simulink model "TypeA_siso180515"  (R2014a)
settings: Solver=ode45  StartTime=0.0  StopTime=12.0  RelTol=1e-3
values from neighbouring files (symbols this model uses):
  gain_actIML = 2.1e-7*1.e+6*20/(2^16)/magIM(inddc)*gain_actIML    [TypeA_reconstruction.m]
  gain_actMNL = 5.1e-6*1.e+6*20/(2^16)/magMN(inddc)*gain_actMNL    [TypeA_reconstruction.m]
  gain_actTML = 1.7e-7*1.e+6*20/(2^16)/magTM(inddc)*gain_actTML    [TypeA_reconstruction.m]
  gainBFL = 0    [main.m]
  gainIPL = 0    [main.m]
  sys1 = sys1_exp    [check_exportvsmake.m]    (also in sumcon2mdlconst_typeA.m = sus.ss)
undefined symbols (not defined in the file or in its folder): cMat_BF, cMat_IM, cMat_MN, cMat_TM, gain_actBFGAS, gain_actBFL, gain_actBFP, gain_actBFR, gain_actBFT, gain_actBFV, gain_actBFY, gain_actF0GAS, gain_actF1GAS, gain_actF2GAS, gain_actF3GAS, gain_actIMP, gain_actIMR, gain_actIMT, gain_actIMV, gain_actIMY, gain_actIPL, gain_actIPT, gain_actIPY, gain_actMNP, gain_actMNR, gain_actMNT, gain_actMNV, gain_actMNY, gain_actTMP, gain_actTMY, gainBFGAS, gainBFP, gainBFR, gainBFT, gainBFV, gainBFY, gainF0GAS, gainF1GAS, gainF2GAS, gainF3GAS, gainHieBFP, gainHieBFR, gainHieBFY, gainHieIML, gainHieIMP, gainHieIMY, gainHieIPL, gainHieIPY, gainHieMNL, gainHieMNP, gainHieMNY, gainIML, gainIMP, gainIMR, gainIMT, gainIMV, gainIMY, gainIPT, gainIPY, gainISC_TML ... (+18)
libraries: cstblocks x57
(part 1 of 2)
settings Model: Creator=kokioktm  LastModifiedBy=ayaka
settings DebuggingCC: MergeDetectMultiDrivingBlocksExec=error  FrameProcessingCompatibilityMsg=error

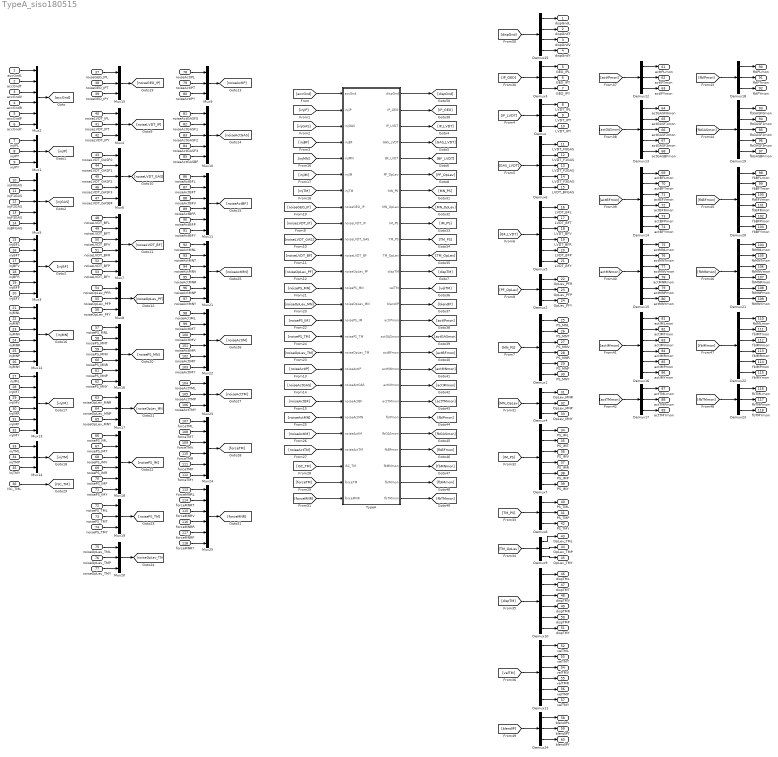
== system TypeA_siso180515 ==
  accGndL : Inport
  accGndT : Inport  Port=2
  accGndV : Inport  Port=3
  accGndR : Inport  Port=4
  accGndP : Inport  Port=5
  accGndY : Inport  Port=6
  injIPL : Inport  Port=7
  injIPT : Inport  Port=8
  injIPY : Inport  Port=9
  injF0GAS : Inport  Port=10
  injF1GAS : Inport  Port=11
  injF2GAS : Inport  Port=12
  injF3GAS : Inport  Port=13
  injBFGAS : Inport  Port=14
  injBFL : Inport  Port=15
  injBFT : Inport  Port=16
  injBFV : Inport  Port=17
  injBFR : Inport  Port=18
  injBFP : Inport  Port=19
  injBFY : Inport  Port=20
  injMNL : Inport  Port=21
  injMNT : Inport  Port=22
  injMNV : Inport  Port=23
  injMNR : Inport  Port=24
  injMNP : Inport  Port=25
  injMNY : Inport  Port=26
  injIML : Inport  Port=27
  injIMT : Inport  Port=28
  injIMV : Inport  Port=29
  injIMR : Inport  Port=30
  injIMP : Inport  Port=31
  injIMY : Inport  Port=32
  injTML : Inport  Port=33
  injTMP : Inport  Port=34
  injTMY : Inport  Port=35
  ISC_TML : Inport  Port=36
  noiseGEO_IPL : Inport  Port=37
  noiseGEO_IPT : Inport  Port=38
  noiseGEO_IPY : Inport  Port=39
  noiseLVDT_IPL : Inport  Port=40
  noiseLVDT_IPT : Inport  Port=41
  noiseLVDT_IPY : Inport  Port=42
  noiseLVDT_GASF0 : Inport  Port=43
  noiseLVDT_GASF1 : Inport  Port=44
  noiseLVDT_GASF2 : Inport  Port=45
  noiseLVDT_GASF3 : Inport  Port=46
  noiseLVDT_GASBF : Inport  Port=47
  noiseLVDT_BFL : Inport  Port=48
  noiseLVDT_BFT : Inport  Port=49
  noiseLVDT_BFV : Inport  Port=50
  noiseLVDT_BFR : Inport  Port=51
  noiseLVDT_BFP : Inport  Port=52
  noiseLVDT_BFY : Inport  Port=53
  noiseOpLev_PFR : Inport  Port=54
  noiseOpLev_PFP : Inport  Port=55
  noiseOpLev_PFY : Inport  Port=56
  noisePS_MNL : Inport  Port=57
  noisePS_MNT : Inport  Port=58
  noisePS_MNV : Inport  Port=59
  noisePS_MNR : Inport  Port=60
  noisePS_MNP : Inport  Port=61
  noisePS_MNY : Inport  Port=62
  noiseOpLev_MNR : Inport  Port=63
  noiseOpLev_MNP : Inport  Port=64
  noiseOpLev_MNY : Inport  Port=65
  noisePS_IML : Inport  Port=66
  noisePS_IMT : Inport  Port=67
  noisePS_IMV : Inport  Port=68
  noisePS_IMR : Inport  Port=69
  noisePS_IMP : Inport  Port=70
  noisePS_IMY : Inport  Port=71
  noisePS_TML : Inport  Port=72
  noisePS_TMT : Inport  Port=73
  noisePS_TMY : Inport  Port=74
  noiseOpLev_TML : Inport  Port=75
  noiseOpLev_TMP : Inport  Port=76
  noiseOpLev_TMY : Inport  Port=77
  noiseActIPL : Inport  Port=78
  noiseActIPT : Inport  Port=79
  noiseActIPY : Inport  Port=80
  noiseActGASF0 : Inport  Port=81
  noiseActGASF1 : Inport  Port=82
  noiseActGASF2 : Inport  Port=83
  noiseActGASF3 : Inport  Port=84
  noiseActGASBF : Inport  Port=85
  noiseActBFL : Inport  Port=86
  noiseActBFT : Inport  Port=87
  noiseActBFV : Inport  Port=88
  noiseActBFR : Inport  Port=89
  noiseActBFP : Inport  Port=90
  noiseActBFY : Inport  Port=91
  noiseActMNL : Inport  Port=92
  noiseActMNT : Inport  Port=93
  noiseActMNV : Inport  Port=94
  noiseActMNR : Inport  Port=95
  noiseActMNP : Inport  Port=96
  noiseActMNY : Inport  Port=97
  noiseActIML : Inport  Port=98
  noiseActIMT : Inport  Port=99
  noiseActIMV : Inport  Port=100
  noiseActIMR : Inport  Port=101
  noiseActIMP : Inport  Port=102
  noiseActIMY : Inport  Port=103
  noiseActTML : Inport  Port=104
  noiseActTMP : Inport  Port=105
  noiseActTMY : Inport  Port=106
  forceTML : Inport  Port=107
  forceTMT : Inport  Port=108
  forceTMV : Inport  Port=109
  forceTMR : Inport  Port=110
  forceTMP : Inport  Port=111
  forceTMY : Inport  Port=112
  forceMNRL : Inport  Port=113
  forceMNRT : Inport  Port=114
  forceMNRV : Inport  Port=115
  forceMNRR : Inport  Port=116
  forceMNRP : Inport  Port=117
  forceMNRY : Inport  Port=118
  Demux{,2..4,8..9,12,17..18,23..24} (11 alike) : Demux  Outputs=3
  Demux{1,5,7,10..11,14..16,20..22} (11 alike) : Demux  Outputs=6
  Demux13 : Demux  Outputs=5
  Demux19 : Demux  Outputs=5
  Demux25 : Demux
  Demux6 : Demux  Outputs=5
  Mux{1,4,8..9,14..15,17,19..20,23} (10 alike) : Mux  Inputs=3
  Mux10 : Mux  Inputs=5
  Mux{2..3,7,11..13,16,18,21..22,24..25} (12 alike) : Mux  Inputs=6
  Mux5 : Mux  Inputs=5
  Mux6 : Mux  Inputs=5
  TypeA : Subsystem
  dispGndL : Outport
  dispGndT : Outport  Port=2
  dispGndV : Outport  Port=3
  dispGndY : Outport  Port=4
  GEO_IPL : Outport  Port=5
  GEO_IPT : Outport  Port=6
  GEO_IPY : Outport  Port=7
  LVDT_IPL : Outport  Port=8
  LVDT_IPT : Outport  Port=9
  LVDT_IPY : Outport  Port=10
  LVDT_F0GAS : Outport  Port=11
  LVDT_F1GAS : Outport  Port=12
  LVDT_F2GAS : Outport  Port=13
  LVDT_F3GAS : Outport  Port=14
  LVDT_BFGAS : Outport  Port=15
  LVDT_BFL : Outport  Port=16
  LVDT_BFT : Outport  Port=17
  LVDT_BFV : Outport  Port=18
  LVDT_BFR : Outport  Port=19
  LVDT_BFP : Outport  Port=20
  LVDT_BFY : Outport  Port=21
  OpLev_PFR : Outport  Port=22
  OpLev_PFP : Outport  Port=23
  OpLev_PFY : Outport  Port=24
  PS_MNL : Outport  Port=25
  PS_MNT : Outport  Port=26
  PS_MNV : Outport  Port=27
  PS_MNR : Outport  Port=28
  PS_MNP : Outport  Port=29
  PS_MNY : Outport  Port=30
  OpLev_MNR : Outport  Port=31
  OpLev_MNP : Outport  Port=32
  OpLev_MNY : Outport  Port=33
  PS_IML : Outport  Port=34
  PS_IMT : Outport  Port=35
  PS_IMV : Outport  Port=36
  PS_IMR : Outport  Port=37
  PS_IMP : Outport  Port=38
  PS_IMY : Outport  Port=39
  PS_TML : Outport  Port=40
  PS_TMP : Outport  Port=41
  PS_TMY : Outport  Port=42
  OpLev_TML : Outport  Port=43
  OpLev_TMP : Outport  Port=44
  OpLev_TMY : Outport  Port=45
  dispTML : Outport  Port=46
  dispTMT : Outport  Port=47
  dispTMV : Outport  Port=48
  dispTMR : Outport  Port=49
  dispTMP : Outport  Port=50
  dispTMY : Outport  Port=51
  velTML : Outport  Port=52
  velTMT : Outport  Port=53
  velTMV : Outport  Port=54
  velTMR : Outport  Port=55
  velTMP : Outport  Port=56
  velTMY : Outport  Port=57
  blendIPL : Outport  Port=58
  blendIPT : Outport  Port=59
  blendIPY : Outport  Port=60
  actIPLmon : Outport  Port=61
  actIPTmon : Outport  Port=62
  actIPYmon : Outport  Port=63
  actGASF0mon : Outport  Port=64
  actGASF1mon : Outport  Port=65
  actGASF2mon : Outport  Port=66
  actGASF3mon : Outport  Port=67
  actGASBFmon : Outport  Port=68
  actBFLmon : Outport  Port=69
  actBFTmon : Outport  Port=70
  actBFVmon : Outport  Port=71
  actBFRmon : Outport  Port=72
  actBFPmon : Outport  Port=73
  actBFYmon : Outport  Port=74
  actMNLmon : Outport  Port=75
  actMNTmon : Outport  Port=76
  actMNVmon : Outport  Port=77
  actMNRmon : Outport  Port=78
  actMNPmon : Outport  Port=79
  actMNYmon : Outport  Port=80
  actIMLmon : Outport  Port=81
  actIMTmon : Outport  Port=82
  actIMVmon : Outport  Port=83
  actIMRmon : Outport  Port=84
  actIMPmon : Outport  Port=85
  actIMYmon : Outport  Port=86
  actTMLmon : Outport  Port=87
  actTMPmon : Outport  Port=88
  actTMYmon : Outport  Port=89
  fbIPLmon : Outport  Port=90
  fbIPTmon : Outport  Port=91
  fbIPYmon : Outport  Port=92
  fbGASF0mon : Outport  Port=93
  fbGASF1mon : Outport  Port=94
  fbGASF2mon : Outport  Port=95
  fbGASF3mon : Outport  Port=96
  fbGASBFmon : Outport  Port=97
  fbBFLmon : Outport  Port=98
  fbBFTmon : Outport  Port=99
  fbBFVmon : Outport  Port=100
  fbBFRmon : Outport  Port=101
  fbBFPmon : Outport  Port=102
  fbBFYmon : Outport  Port=103
  fbMNLmon : Outport  Port=104
  fbMNTmon : Outport  Port=105
  fbMNVmon : Outport  Port=106
  fbMNRmon : Outport  Port=107
  fbMNPmon : Outport  Port=108
  fbMNYmon : Outport  Port=109
  fbIMLmon : Outport  Port=110
  fbIMTmon : Outport  Port=111
  fbIMVmon : Outport  Port=112
  fbIMRmon : Outport  Port=113
  fbIMPmon : Outport  Port=114
  fbIMYmon : Outport  Port=115
  fbTMLmon : Outport  Port=116
  fbTMPmon : Outport  Port=117
  fbTMYmon : Outport  Port=118
  wires:
  [accGnd] -> TypeA/1(accGnd)
  accGndT/1 -> Mux2/2
  accGndL/1 -> Mux2/1
  accGndV/1 -> Mux2/3
  accGndR/1 -> Mux2/4
  accGndP/1 -> Mux2/5
  accGndY/1 -> Mux2/6
  Mux2/1 -> [accGnd]
  injIPL/1 -> Mux1/1
  injIPT/1 -> Mux1/2
  injIPY/1 -> Mux1/3
  Mux1/1 -> [injIP]
  [injIP] -> TypeA/2(injIP)
  injF0GAS/1 -> Mux5/1
  injF1GAS/1 -> Mux5/2
  injF2GAS/1 -> Mux5/3
  injF3GAS/1 -> Mux5/4
  injBFGAS/1 -> Mux5/5
  Mux5/1 -> [injGAS]
  [injGAS] -> TypeA/3(injGAS)
  injBFT/1 -> Mux3/2
  injBFL/1 -> Mux3/1
  injBFV/1 -> Mux3/3
  injBFR/1 -> Mux3/4
  injBFP/1 -> Mux3/5
  injBFY/1 -> Mux3/6
  Mux3/1 -> [injBF]
  [injBF] -> TypeA/4(injBF)
  TypeA/3(IP_LVDT) -> [IP_LVDT]
  TypeA/4(GAS_LVDT) -> [GAS_LVDT]
  TypeA/5(BF_LVDT) -> [BF_LVDT]
  TypeA/12(dispTM) -> [dispTM]
  TypeA/6(PF_OpLev) -> [PF_OpLev]
  [IP_LVDT] -> Demux/1
  Demux/1 -> LVDT_IPL/1
  Demux/2 -> LVDT_IPT/1
  Demux/3 -> LVDT_IPY/1
  [GAS_LVDT] -> Demux6/1
  Demux6/1 -> LVDT_F0GAS/1
  Demux6/2 -> LVDT_F1GAS/1
  Demux6/3 -> LVDT_F2GAS/1
  Demux6/4 -> LVDT_F3GAS/1
  Demux6/5 -> LVDT_BFGAS/1
  [BF_LVDT] -> Demux5/1
  Demux5/1 -> LVDT_BFL/1
  Demux5/2 -> LVDT_BFT/1
  Demux5/3 -> LVDT_BFV/1
  Demux5/4 -> LVDT_BFR/1
  Demux5/5 -> LVDT_BFP/1
  Demux5/6 -> LVDT_BFY/1
  Demux1/1 -> PS_MNL/1
  Demux1/2 -> PS_MNT/1
  Demux1/3 -> PS_MNV/1
  Demux1/4 -> PS_MNR/1
  Demux1/5 -> PS_MNP/1
  Demux1/6 -> PS_MNY/1
  [MN_PS] -> Demux1/1
  [PF_OpLev] -> Demux2/1
  Demux2/2 -> OpLev_PFP/1
  Demux2/3 -> OpLev_PFY/1
  noiseLVDT_IPL/1 -> Mux4/1
  noiseLVDT_IPT/1 -> Mux4/2
  noiseLVDT_IPY/1 -> Mux4/3
  Mux4/1 -> [noiseLVDT_IP]
  noiseLVDT_GASF0/1 -> Mux6/1
  noiseLVDT_GASF1/1 -> Mux6/2
  noiseLVDT_GASF2/1 -> Mux6/3
  noiseLVDT_GASF3/1 -> Mux6/4
  noiseLVDT_GASBF/1 -> Mux6/5
  Mux6/1 -> [noiseLVDT_GAS]
  noiseLVDT_BFT/1 -> Mux7/2
  noiseLVDT_BFL/1 -> Mux7/1
  noiseLVDT_BFV/1 -> Mux7/3
  noiseLVDT_BFR/1 -> Mux7/4
  noiseLVDT_BFP/1 -> Mux7/5
  noiseLVDT_BFY/1 -> Mux7/6
  Mux7/1 -> [noiseLVDT_BF]
  noiseOpLev_PFR/1 -> Mux8/1
  noiseOpLev_PFP/1 -> Mux8/2
  Mux8/1 -> [noiseOpLev_PF]
  [noiseLVDT_IP] -> TypeA/9(noiseLVDT_IP)
  [noiseLVDT_GAS] -> TypeA/10(noiseLVDT_GAS)
  [noiseOpLev_PF] -> TypeA/12(noiseOpLev_PF)
  [noiseLVDT_BF] -> TypeA/11(noiseLVDT_BF)
  noiseActIPL/1 -> Mux9/1
  noiseActIPT/1 -> Mux9/2
  noiseActIPY/1 -> Mux9/3
  Mux9/1 -> [noiseActIP]
  noiseActGASF0/1 -> Mux10/1
  noiseActGASF1/1 -> Mux10/2
  noiseActGASF2/1 -> Mux10/3
  noiseActGASF3/1 -> Mux10/4
  noiseActGASBF/1 -> Mux10/5
  Mux10/1 -> [noiseActGAS]
  noiseActBFT/1 -> Mux11/2
  noiseActBFL/1 -> Mux11/1
  noiseActBFV/1 -> Mux11/3
  noiseActBFR/1 -> Mux11/4
  noiseActBFP/1 -> Mux11/5
  noiseActBFY/1 -> Mux11/6
  Mux11/1 -> [noiseActBF]
  [noiseActGAS] -> TypeA/19(noiseActGAS)
  [noiseActBF] -> TypeA/20(noiseActBF)
  [noiseActIP] -> TypeA/18(noiseActIP)
  [injMN] -> TypeA/5(injMN)
  [injTM] -> TypeA/7(injTM)
  [injIM] -> TypeA/6(injIM)
  injMNT/1 -> Mux12/2
  injMNL/1 -> Mux12/1
  injMNV/1 -> Mux12/3
  injMNR/1 -> Mux12/4
  injMNP/1 -> Mux12/5
  injMNY/1 -> Mux12/6
  Mux12/1 -> [injMN]
  injIMT/1 -> Mux13/2
  injIML/1 -> Mux13/1
  injIMV/1 -> Mux13/3
  injIMR/1 -> Mux13/4
  injIMP/1 -> Mux13/5
  injIMY/1 -> Mux13/6
  Mux13/1 -> [injIM]
  injTML/1 -> Mux14/1
  injTMP/1 -> Mux14/2
  injTMY/1 -> Mux14/3
  Mux14/1 -> [injTM]
  noiseGEO_IPL/1 -> Mux15/1
  noiseGEO_IPT/1 -> Mux15/2
  noiseGEO_IPY/1 -> Mux15/3
  Mux15/1 -> [noiseGEO_IP]
  [noiseGEO_IP] -> TypeA/8(noiseGEO_IP)
  noiseOpLev_PFY/1 -> Mux8/3
  noisePS_MNT/1 -> Mux16/2
  noisePS_MNL/1 -> Mux16/1
  noisePS_MNV/1 -> Mux16/3
  noisePS_MNR/1 -> Mux16/4
  noisePS_MNP/1 -> Mux16/5
  noisePS_MNY/1 -> Mux16/6
  Mux16/1 -> [noisePS_MN]
  noiseOpLev_MNR/1 -> Mux17/1
  noiseOpLev_MNP/1 -> Mux17/2
  Mux17/1 -> [noiseOpLev_MN]
  noiseOpLev_MNY/1 -> Mux17/3
  noisePS_IMT/1 -> Mux18/2
  noisePS_IML/1 -> Mux18/1
  noisePS_IMV/1 -> Mux18/3
  noisePS_IMR/1 -> Mux18/4
  noisePS_IMP/1 -> Mux18/5
  noisePS_IMY/1 -> Mux18/6
  Mux18/1 -> [noisePS_IM]
  noisePS_TML/1 -> Mux19/1
  noisePS_TMT/1 -> Mux19/2
  Mux19/1 -> [noisePS_TM]
  noisePS_TMY/1 -> Mux19/3
  noiseOpLev_TMP/1 -> Mux20/2
  noiseOpLev_TMY/1 -> Mux20/3
  Mux20/1 -> [noiseOpLev_TM]
  [noisePS_MN] -> TypeA/13(noisePS_MN)
  [noisePS_IM] -> TypeA/15(noisePS_IM)
  [noiseOpLev_MN] -> TypeA/14(noiseOpLev_MN)
  [noisePS_TM] -> TypeA/16(noisePS_TM)
  [noiseOpLev_TM] -> TypeA/17(noiseOpLev_TM)
  noiseActMNT/1 -> Mux21/2
  noiseActMNL/1 -> Mux21/1
  noiseActMNV/1 -> Mux21/3
  noiseActMNR/1 -> Mux21/4
  noiseActMNP/1 -> Mux21/5
  noiseActMNY/1 -> Mux21/6
  Mux21/1 -> [noiseActMN]
  noiseActIMT/1 -> Mux22/2
  noiseActIML/1 -> Mux22/1
  noiseActIMV/1 -> Mux22/3
  noiseActIMR/1 -> Mux22/4
  noiseActIMP/1 -> Mux22/5
  noiseActIMY/1 -> Mux22/6
  Mux22/1 -> [noiseActIM]
  noiseActTML/1 -> Mux23/1
  noiseActTMP/1 -> Mux23/2
  noiseActTMY/1 -> Mux23/3
  Mux23/1 -> [noiseActTM]
  forceTMT/1 -> Mux24/2
  forceTML/1 -> Mux24/1
  forceTMV/1 -> Mux24/3
  forceTMR/1 -> Mux24/4
  forceTMP/1 -> Mux24/5
  forceTMY/1 -> Mux24/6
  Mux24/1 -> [forceTM]
  ISC_TML/1 -> [ISC_TM]
  [noiseActMN] -> TypeA/21(noiseActMN)
  [noiseActTM] -> TypeA/23(noiseActTM)
  [noiseActIM] -> TypeA/22(noiseActIM)
  [forceTM] -> TypeA/25(forceTM)
  [ISC_TM] -> TypeA/24(ISC_TM)
  [IP_GEO] -> Demux3/1
  Demux3/1 -> GEO_IPL/1
  Demux3/2 -> GEO_IPT/1
  Demux3/3 -> GEO_IPY/1
  TypeA/2(IP_GEO) -> [IP_GEO]
  Demux2/1 -> OpLev_PFR/1
  TypeA/9(IM_PS) -> [IM_PS]
  TypeA/10(TM_PS) -> [TM_PS]
  TypeA/8(MN_OpLev) -> [MN_OpLev]
  TypeA/7(MN_PS) -> [MN_PS]
  TypeA/11(TM_OpLev) -> [TM_OpLev]
  TypeA/22(fbGASmon) -> [fbGASmon]
  TypeA/16(actGASmon) -> [actGASmon]
  TypeA/21(fbIPmon) -> [fbIPmon]
  TypeA/26(fbTMmon) -> [fbTMmon]
  TypeA/24(fbMNmon) -> [fbMNmon]
  TypeA/15(actIPmon) -> [actIPmon]
  TypeA/19(actIMmon) -> [actIMmon]
  TypeA/14(blendIP) -> [blendIP]
  TypeA/13(velTM) -> [velTM]
  TypeA/25(fbIMmon) -> [fbIMmon]
  TypeA/18(actMNmon) -> [actMNmon]
  TypeA/20(actTMmon) -> [actTMmon]
  TypeA/17(actBFmon) -> [actBFmon]
  TypeA/23(fbBFmon) -> [fbBFmon]
  [MN_OpLev] -> Demux4/1
  Demux4/2 -> OpLev_MNP/1
  Demux4/3 -> OpLev_MNY/1
  Demux4/1 -> OpLev_MNR/1
  Demux7/1 -> PS_IML/1
  Demux7/2 -> PS_IMT/1
  Demux7/3 -> PS_IMV/1
  Demux7/4 -> PS_IMR/1
  Demux7/5 -> PS_IMP/1
  Demux7/6 -> PS_IMY/1
  [IM_PS] -> Demux7/1
  Demux8/1 -> PS_TML/1
  [TM_PS] -> Demux8/1
  Demux8/2 -> PS_TMP/1
  Demux8/3 -> PS_TMY/1
  [TM_OpLev] -> Demux9/1
  Demux10/1 -> dispTML/1
  Demux10/2 -> dispTMT/1
  Demux10/3 -> dispTMV/1
  Demux10/4 -> dispTMR/1
  Demux10/5 -> dispTMP/1
  Demux10/6 -> dispTMY/1
  [dispTM] -> Demux10/1
  Demux11/1 -> velTML/1
  Demux11/2 -> velTMT/1
  Demux11/3 -> velTMV/1
  Demux11/4 -> velTMR/1
  Demux11/5 -> velTMP/1
  Demux11/6 -> velTMY/1
  [velTM] -> Demux11/1
  [actIPmon] -> Demux12/1
  Demux12/1 -> actIPLmon/1
  Demux12/2 -> actIPTmon/1
  Demux12/3 -> actIPYmon/1
  [actGASmon] -> Demux13/1
  Demux13/1 -> actGASF0mon/1
  Demux13/2 -> actGASF1mon/1
  Demux13/3 -> actGASF2mon/1
  Demux13/4 -> actGASF3mon/1
  Demux13/5 -> actGASBFmon/1
  [actBFmon] -> Demux14/1
  Demux14/1 -> actBFLmon/1
  Demux14/2 -> actBFTmon/1
  Demux14/3 -> actBFVmon/1
  Demux14/4 -> actBFRmon/1
  Demux14/5 -> actBFPmon/1
  Demux14/6 -> actBFYmon/1
  [actMNmon] -> Demux15/1
  Demux15/1 -> actMNLmon/1
  Demux15/2 -> actMNTmon/1
  Demux15/3 -> actMNVmon/1
  Demux15/4 -> actMNRmon/1
  Demux15/5 -> actMNPmon/1
  Demux15/6 -> actMNYmon/1
  [actIMmon] -> Demux16/1
  Demux16/1 -> actIMLmon/1
  Demux16/2 -> actIMTmon/1
  Demux16/3 -> actIMVmon/1
  Demux16/4 -> actIMRmon/1
  Demux16/5 -> actIMPmon/1
  Demux16/6 -> actIMYmon/1
  [actTMmon] -> Demux17/1
  Demux17/2 -> actTMPmon/1
  Demux17/3 -> actTMYmon/1
  Demux17/1 -> actTMLmon/1
  [fbIPmon] -> Demux18/1
  Demux18/1 -> fbIPLmon/1
  Demux18/2 -> fbIPTmon/1
  Demux18/3 -> fbIPYmon/1
  [fbGASmon] -> Demux19/1
  Demux19/1 -> fbGASF0mon/1
  Demux19/2 -> fbGASF1mon/1
  Demux19/3 -> fbGASF2mon/1
  Demux19/4 -> fbGASF3mon/1
  Demux19/5 -> fbGASBFmon/1
  [fbBFmon] -> Demux20/1
  Demux20/1 -> fbBFLmon/1
  Demux20/2 -> fbBFTmon/1
  Demux20/3 -> fbBFVmon/1
  Demux20/4 -> fbBFRmon/1
  Demux20/5 -> fbBFPmon/1
  Demux20/6 -> fbBFYmon/1
  [fbMNmon] -> Demux21/1
  Demux21/1 -> fbMNLmon/1
  Demux21/2 -> fbMNTmon/1
  Demux21/3 -> fbMNVmon/1
  Demux21/4 -> fbMNRmon/1
  Demux21/5 -> fbMNPmon/1
  Demux21/6 -> fbMNYmon/1
  [fbIMmon] -> Demux22/1
  Demux22/1 -> fbIMLmon/1
  Demux22/2 -> fbIMTmon/1
  Demux22/3 -> fbIMVmon/1
  Demux22/4 -> fbIMRmon/1
  Demux22/5 -> fbIMPmon/1
  Demux22/6 -> fbIMYmon/1
  [fbTMmon] -> Demux23/1
  Demux23/2 -> fbTMPmon/1
  Demux23/3 -> fbTMYmon/1
  Demux23/1 -> fbTMLmon/1
  Demux24/1 -> blendIPL/1
  [blendIP] -> Demux24/1
  Demux24/2 -> blendIPT/1
  Demux24/3 -> blendIPY/1
  [dispGnd] -> Demux25/1
  Demux25/1 -> dispGndL/1
  Demux25/2 -> dispGndT/1
  Demux25/3 -> dispGndV/1
  Demux25/4 -> dispGndY/1
  TypeA/1(dispGnd) -> [dispGnd]
  forceMNRR/1 -> Mux25/4
  forceMNRP/1 -> Mux25/5
  forceMNRL/1 -> Mux25/1
  forceMNRT/1 -> Mux25/2
  Mux25/1 -> [forceMNR]
  forceMNRV/1 -> Mux25/3
  forceMNRY/1 -> Mux25/6
  [forceMNR] -> TypeA/26(forceMNR)
  noiseOpLev_TML/1 -> Mux20/1
  Demux9/1 -> OpLev_TML/1
  Demux9/2 -> OpLev_TMP/1
  Demux9/3 -> OpLev_TMY/1

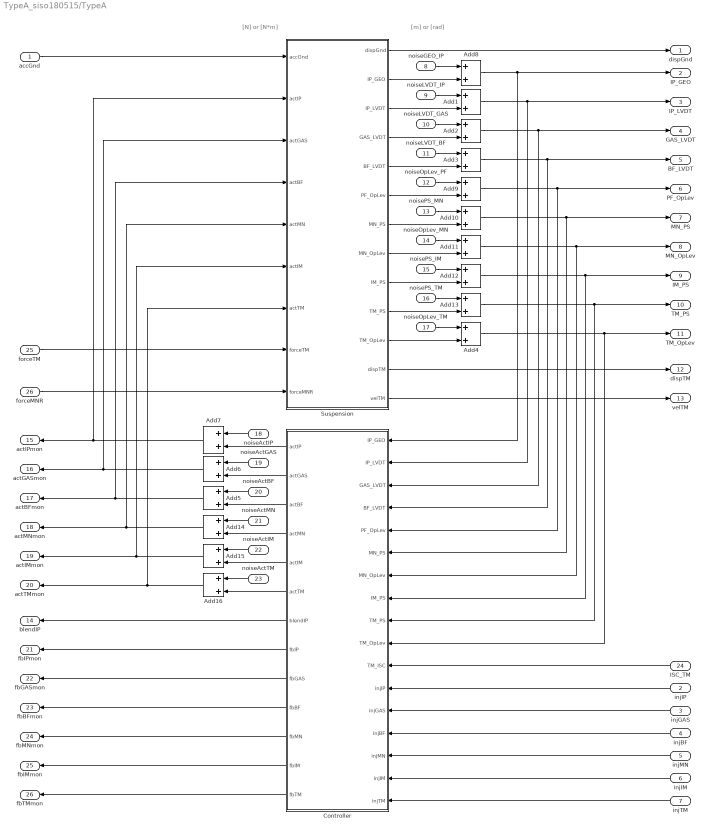
== system TypeA_siso180515/TypeA ==
  note: [N] or [N*m]
  note: [m] or [rad]
  accGnd : Inport
  injIP : Inport  Port=2
  injGAS : Inport  Port=3
  injBF : Inport  Port=4
  injMN : Inport  Port=5
  injIM : Inport  Port=6
  injTM : Inport  Port=7
  noiseGEO_IP : Inport  Port=8
  noiseLVDT_IP : Inport  Port=9
  noiseLVDT_GAS : Inport  Port=10
  noiseLVDT_BF : Inport  Port=11
  noiseOpLev_PF : Inport  Port=12
  noisePS_MN : Inport  Port=13
  noiseOpLev_MN : Inport  Port=14
  noisePS_IM : Inport  Port=15
  noisePS_TM : Inport  Port=16
  noiseOpLev_TM : Inport  Port=17
  noiseActIP : Inport  Port=18
  noiseActGAS : Inport  Port=19
  noiseActBF : Inport  Port=20
  noiseActMN : Inport  Port=21
  noiseActIM : Inport  Port=22
  noiseActTM : Inport  Port=23
  ISC_TM : Inport  Port=24
  forceTM : Inport  Port=25
  forceMNR : Inport  Port=26
  Add{1..16} (16 alike) : Sum
  Controller : Subsystem
  Suspension : Subsystem
  dispGnd : Outport
  IP_GEO : Outport  Port=2
  IP_LVDT : Outport  Port=3
  GAS_LVDT : Outport  Port=4
  BF_LVDT : Outport  Port=5
  PF_OpLev : Outport  Port=6
  MN_PS : Outport  Port=7
  MN_OpLev : Outport  Port=8
  IM_PS : Outport  Port=9
  TM_PS : Outport  Port=10
  TM_OpLev : Outport  Port=11
  dispTM : Outport  Port=12
  velTM : Outport  Port=13
  blendIP : Outport  Port=14
  actIPmon : Outport  Port=15
  actGASmon : Outport  Port=16
  actBFmon : Outport  Port=17
  actMNmon : Outport  Port=18
  actIMmon : Outport  Port=19
  actTMmon : Outport  Port=20
  fbIPmon : Outport  Port=21
  fbGASmon : Outport  Port=22
  fbBFmon : Outport  Port=23
  fbMNmon : Outport  Port=24
  fbIMmon : Outport  Port=25
  fbTMmon : Outport  Port=26
  wires:
  Add1/1 -> IP_LVDT/1, Controller/2(IP_LVDT)
  Add3/1 -> Controller/4(BF_LVDT), BF_LVDT/1
  Add2/1 -> GAS_LVDT/1, Controller/3(GAS_LVDT)
  Suspension/12(dispTM) -> dispTM/1
  Add7/1 -> actIPmon/1, Suspension/2(actIP)
  Add5/1 -> actBFmon/1, Suspension/4(actBF)
  Add4/1 -> Controller/10(TM_OpLev), TM_OpLev/1
  accGnd/1 -> Suspension/1(accGnd)
  Add6/1 -> actGASmon/1, Suspension/3(actGAS)
  injGAS/1 -> Controller/13(injGAS)
  injIP/1 -> Controller/12(injIP)
  injBF/1 -> Controller/14(injBF)
  Controller/10(fbBF) -> fbBFmon/1
  Controller/8(fbIP) -> fbIPmon/1
  Controller/9(fbGAS) -> fbGASmon/1
  Suspension/3(IP_LVDT) -> Add1/2
  Suspension/4(GAS_LVDT) -> Add2/2
  Suspension/5(BF_LVDT) -> Add3/2
  Suspension/11(TM_OpLev) -> Add4/2
  noiseLVDT_IP/1 -> Add1/1
  noiseLVDT_GAS/1 -> Add2/1
  noiseLVDT_BF/1 -> Add3/1
  noiseOpLev_TM/1 -> Add4/1
  Controller/3(actBF) -> Add5/2
  Controller/1(actIP) -> Add7/2
  Controller/2(actGAS) -> Add6/2
  noiseActIP/1 -> Add7/1
  noiseActGAS/1 -> Add6/1
  noiseActBF/1 -> Add5/1
  Add8/1 -> Controller/1(IP_GEO), IP_GEO/1
  noiseGEO_IP/1 -> Add8/1
  Suspension/2(IP_GEO) -> Add8/2
  noiseOpLev_PF/1 -> Add9/1
  Suspension/6(PF_OpLev) -> Add9/2
  Add9/1 -> Controller/5(PF_OpLev), PF_OpLev/1
  noisePS_MN/1 -> Add10/1
  Add10/1 -> Controller/6(MN_PS), MN_PS/1
  noiseOpLev_MN/1 -> Add11/1
  Add11/1 -> Controller/7(MN_OpLev), MN_OpLev/1
  noisePS_IM/1 -> Add12/1
  Add12/1 -> Controller/8(IM_PS), IM_PS/1
  Suspension/8(MN_OpLev) -> Add11/2
  Suspension/7(MN_PS) -> Add10/2
  Suspension/9(IM_PS) -> Add12/2
  noisePS_TM/1 -> Add13/1
  Add13/1 -> Controller/9(TM_PS), TM_PS/1
  Suspension/10(TM_PS) -> Add13/2
  Suspension/13(velTM) -> velTM/1
  injMN/1 -> Controller/15(injMN)
  injTM/1 -> Controller/17(injTM)
  injIM/1 -> Controller/16(injIM)
  ISC_TM/1 -> Controller/11(TM_ISC)
  noiseActMN/1 -> Add14/1
  Add14/1 -> Suspension/5(actMN), actMNmon/1
  Controller/4(actMN) -> Add14/2
  noiseActIM/1 -> Add15/1
  Add15/1 -> Suspension/6(actIM), actIMmon/1
  Controller/5(actIM) -> Add15/2
  noiseActTM/1 -> Add16/1
  Add16/1 -> Suspension/7(actTM), actTMmon/1
  Controller/6(actTM) -> Add16/2
  Controller/7(blendIP) -> blendIP/1
  Controller/13(fbTM) -> fbTMmon/1
  Controller/11(fbMN) -> fbMNmon/1
  Controller/12(fbIM) -> fbIMmon/1
  forceTM/1 -> Suspension/8(forceTM)
  Suspension/1(dispGnd) -> dispGnd/1
  forceMNR/1 -> Suspension/9(forceMNR)

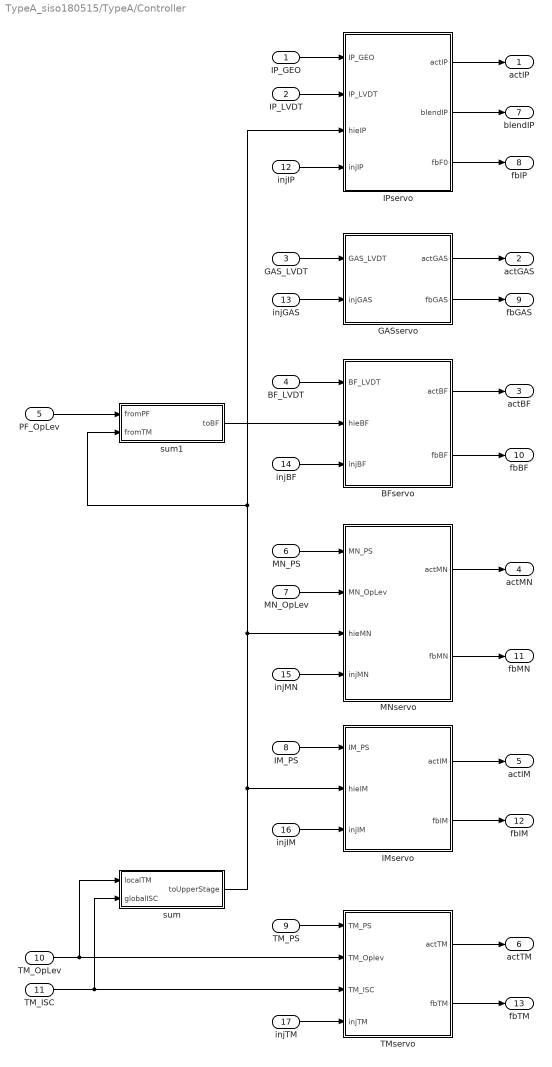
== system TypeA_siso180515/TypeA/Controller ==
  IP_GEO : Inport
  IP_LVDT : Inport  Port=2
  GAS_LVDT : Inport  Port=3
  BF_LVDT : Inport  Port=4
  PF_OpLev : Inport  Port=5
  MN_PS : Inport  Port=6
  MN_OpLev : Inport  Port=7
  IM_PS : Inport  Port=8
  TM_PS : Inport  Port=9
  TM_OpLev : Inport  Port=10
  TM_ISC : Inport  Port=11
  injIP : Inport  Port=12
  injGAS : Inport  Port=13
  injBF : Inport  Port=14
  injMN : Inport  Port=15
  injIM : Inport  Port=16
  injTM : Inport  Port=17
  BFservo : Subsystem
  GASservo : Subsystem
  IMservo : Subsystem
  IPservo : Subsystem
  MNservo : Subsystem
  TMservo : Subsystem
  sum : Subsystem
  sum1 : Subsystem
  actIP : Outport
  actGAS : Outport  Port=2
  actBF : Outport  Port=3
  actMN : Outport  Port=4
  actIM : Outport  Port=5
  actTM : Outport  Port=6
  blendIP : Outport  Port=7
  fbIP : Outport  Port=8
  fbGAS : Outport  Port=9
  fbBF : Outport  Port=10
  fbMN : Outport  Port=11
  fbIM : Outport  Port=12
  fbTM : Outport  Port=13
  wires:
  IP_LVDT/1 -> IPservo/2(IP_LVDT)
  injIP/1 -> IPservo/4(injIP)
  IPservo/3(fbF0) -> fbIP/1
  IPservo/1(actIP) -> actIP/1
  GASservo/1(actGAS) -> actGAS/1
  GASservo/2(fbGAS) -> fbGAS/1
  GAS_LVDT/1 -> GASservo/1(GAS_LVDT)
  injGAS/1 -> GASservo/2(injGAS)
  BF_LVDT/1 -> BFservo/1(BF_LVDT)
  injBF/1 -> BFservo/3(injBF)
  BFservo/1(actBF) -> actBF/1
  BFservo/2(fbBF) -> fbBF/1
  IP_GEO/1 -> IPservo/1(IP_GEO)
  IPservo/2(blendIP) -> blendIP/1
  TM_ISC/1 -> sum/2(globalISC), TMservo/3(TM_ISC)
  TM_OpLev/1 -> sum/1(localTM), TMservo/2(TM_Oplev)
  TM_PS/1 -> TMservo/1(TM_PS)
  injTM/1 -> TMservo/4(injTM)
  MN_PS/1 -> MNservo/1(MN_PS)
  MN_OpLev/1 -> MNservo/2(MN_OpLev)
  injMN/1 -> MNservo/4(injMN)
  IM_PS/1 -> IMservo/1(IM_PS)
  injIM/1 -> IMservo/3(injIM)
  TMservo/1(actTM) -> actTM/1
  TMservo/2(fbTM) -> fbTM/1
  IMservo/2(fbIM) -> fbIM/1
  IMservo/1(actIM) -> actIM/1
  MNservo/2(fbMN) -> fbMN/1
  MNservo/1(actMN) -> actMN/1
  sum/1(toUpperStage) -> sum1/2(fromTM), IPservo/3(hieIP), MNservo/3(hieMN), IMservo/2(hieIM)
  sum1/1(toBF) -> BFservo/2(hieBF)
  PF_OpLev/1 -> sum1/1(fromPF)

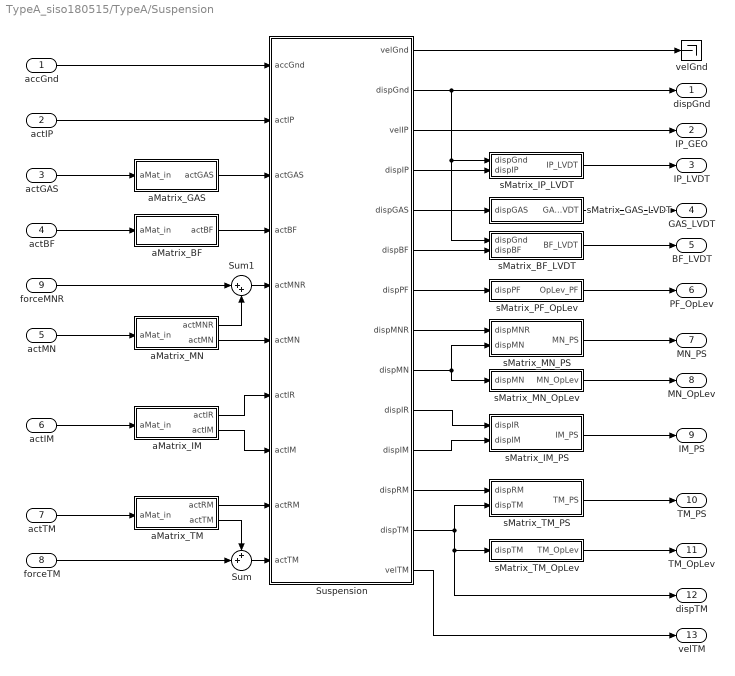
== system TypeA_siso180515/TypeA/Suspension ==
  accGnd : Inport
  actIP : Inport  Port=2
  actGAS : Inport  Port=3
  actBF : Inport  Port=4
  actMN : Inport  Port=5
  actIM : Inport  Port=6
  actTM : Inport  Port=7
  forceTM : Inport  Port=8
  forceMNR : Inport  Port=9
  Sum : Sum  Inputs=++|
  Sum1 : Sum  Inputs=|++
  Suspension : Subsystem
  aMatrix_BF : Subsystem
  aMatrix_GAS : Subsystem
  aMatrix_IM : Subsystem
  aMatrix_MN : Subsystem
  aMatrix_TM : Subsystem
  sMatrix_BF_LVDT : Subsystem
  sMatrix_GAS_LVDT : Subsystem
  sMatrix_IM_PS : Subsystem
  sMatrix_IP_LVDT : Subsystem
  sMatrix_MN_OpLev : Subsystem
  sMatrix_MN_PS : Subsystem
  sMatrix_PF_OpLev : Subsystem
  sMatrix_TM_OpLev : Subsystem
  sMatrix_TM_PS : Subsystem
  velGnd : Terminator
  dispGnd : Outport
  IP_GEO : Outport  Port=2
  IP_LVDT : Outport  Port=3
  GAS_LVDT : Outport  Port=4
  BF_LVDT : Outport  Port=5
  PF_OpLev : Outport  Port=6
  MN_PS : Outport  Port=7
  MN_OpLev : Outport  Port=8
  IM_PS : Outport  Port=9
  TM_PS : Outport  Port=10
  TM_OpLev : Outport  Port=11
  dispTM : Outport  Port=12
  velTM : Outport  Port=13
  wires:
  Suspension/2(dispGnd) -> dispGnd/1, sMatrix_BF_LVDT/1(dispGnd), sMatrix_IP_LVDT/1(dispGnd)
  Suspension/4(dispIP) -> sMatrix_IP_LVDT/2(dispIP)
  Suspension/5(dispGAS) -> sMatrix_GAS_LVDT/1(dispGAS)
  Suspension/6(dispBF) -> sMatrix_BF_LVDT/2(dispBF)
  Suspension/1(velGnd) -> velGnd/1
  sMatrix_IP_LVDT/1(IP_LVDT) -> IP_LVDT/1
  sMatrix_GAS_LVDT/1(GAS_LVDT) -> GAS_LVDT/1
  sMatrix_BF_LVDT/1(BF_LVDT) -> BF_LVDT/1
  Suspension/13(dispTM) -> dispTM/1, sMatrix_TM_OpLev/1(dispTM), sMatrix_TM_PS/2(dispTM)
  accGnd/1 -> Suspension/1(accGnd)
  actIP/1 -> Suspension/2(actIP)
  actGAS/1 -> aMatrix_GAS/1(aMat_in)
  actBF/1 -> aMatrix_BF/1(aMat_in)
  sMatrix_TM_OpLev/1(TM_OpLev) -> TM_OpLev/1
  aMatrix_GAS/1(actGAS) -> Suspension/3(actGAS)
  aMatrix_BF/1(actBF) -> Suspension/4(actBF)
  Suspension/7(dispPF) -> sMatrix_PF_OpLev/1(dispPF)
  sMatrix_PF_OpLev/1(OpLev_PF) -> PF_OpLev/1
  Suspension/8(dispMNR) -> sMatrix_MN_PS/1(dispMNR)
  Suspension/9(dispMN) -> sMatrix_MN_PS/2(dispMN), sMatrix_MN_OpLev/1(dispMN)
  sMatrix_MN_PS/1(MN_PS) -> MN_PS/1
  sMatrix_MN_OpLev/1(MN_OpLev) -> MN_OpLev/1
  Suspension/10(dispIR) -> sMatrix_IM_PS/1(dispIR)
  Suspension/11(dispIM) -> sMatrix_IM_PS/2(dispIM)
  sMatrix_IM_PS/1(IM_PS) -> IM_PS/1
  Suspension/12(dispRM) -> sMatrix_TM_PS/1(dispRM)
  sMatrix_TM_PS/1(TM_PS) -> TM_PS/1
  Suspension/14(velTM) -> velTM/1
  aMatrix_MN/1(actMNR) -> Sum1/2
  aMatrix_MN/2(actMN) -> Suspension/6(actMN)
  actMN/1 -> aMatrix_MN/1(aMat_in)
  actIM/1 -> aMatrix_IM/1(aMat_in)
  aMatrix_IM/1(actIR) -> Suspension/7(actIR)
  aMatrix_IM/2(actIM) -> Suspension/8(actIM)
  actTM/1 -> aMatrix_TM/1(aMat_in)
  aMatrix_TM/1(actRM) -> Suspension/9(actRM)
  Sum/1 -> Suspension/10(actTM)
  aMatrix_TM/2(actTM) -> Sum/1
  forceTM/1 -> Sum/2
  Suspension/3(velIP) -> IP_GEO/1
  Sum1/1 -> Suspension/5(actMNR)
  forceMNR/1 -> Sum1/1

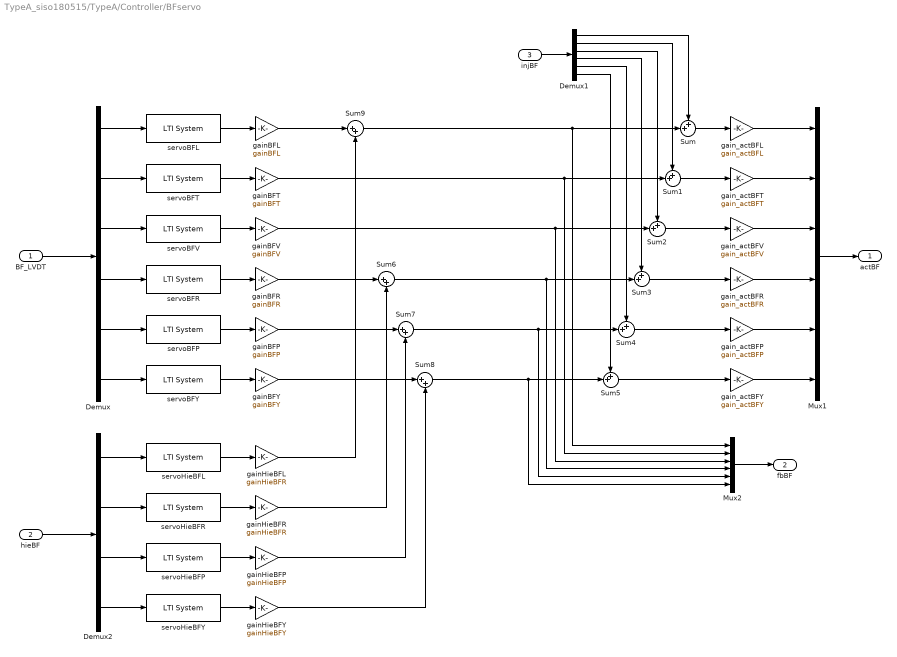
== system TypeA_siso180515/TypeA/Controller/BFservo ==
  BF_LVDT : Inport
  hieBF : Inport  Port=2
  injBF : Inport  Port=3
  Demux : Demux  Outputs=6
  Demux1 : Demux  Outputs=6
  Demux2 : Demux
  Mux1 : Mux  Inputs=6
  Mux2 : Mux  Inputs=6
  Sum{,1..5} (6 alike) : Sum  Inputs=++|
  Sum{6..9} (4 alike) : Sum  Inputs=|++
  gainBFL : Gain  Gain=gainBFL
  gainBFP : Gain  Gain=gainBFP
  gainBFR : Gain  Gain=gainBFR
  gainBFT : Gain  Gain=gainBFT
  gainBFV : Gain  Gain=gainBFV
  gainBFY : Gain  Gain=gainBFY
  gainHieBFL : Gain  Gain=gainHieBFR
  gainHieBFP : Gain  Gain=gainHieBFP
  gainHieBFR : Gain  Gain=gainHieBFR
  gainHieBFY : Gain  Gain=gainHieBFY
  gain_actBFL : Gain  Gain=gain_actBFL
  gain_actBFP : Gain  Gain=gain_actBFP
  gain_actBFR : Gain  Gain=gain_actBFR
  gain_actBFT : Gain  Gain=gain_actBFT
  gain_actBFV : Gain  Gain=gain_actBFV
  gain_actBFY : Gain  Gain=gain_actBFY
  servoBFL : cstblocks/LTI System  sys=servoBFL  IC=[]
  servoBFP : cstblocks/LTI System  sys=servoBFP  IC=[]
  servoBFR : cstblocks/LTI System  sys=servoBFR  IC=[]
  servoBFT : cstblocks/LTI System  sys=servoBFT  IC=[]
  servoBFV : cstblocks/LTI System  sys=servoBFV  IC=[]
  servoBFY : cstblocks/LTI System  sys=servoBFY  IC=[]
  servoHieBFL : cstblocks/LTI System  sys=servoHieBFL  IC=[]
  servoHieBFP : cstblocks/LTI System  sys=servoHieBFP  IC=[]
  servoHieBFR : cstblocks/LTI System  sys=servoHieBFR  IC=[]
  servoHieBFY : cstblocks/LTI System  sys=servoHieBFY  IC=[]
  actBF : Outport
  fbBF : Outport  Port=2
  wires:
  BF_LVDT/1 -> Demux/1
  servoBFL/1 -> gainBFL/1
  servoBFT/1 -> gainBFT/1
  servoBFV/1 -> gainBFV/1
  Demux/1 -> servoBFL/1
  Demux/2 -> servoBFT/1
  Demux/3 -> servoBFV/1
  Sum9/1 -> Sum/2, Mux2/1
  gainBFT/1 -> Sum1/2, Mux2/2
  gainBFV/1 -> Sum2/2, Mux2/3
  injBF/1 -> Demux1/1
  Sum1/1 -> gain_actBFT/1
  Sum2/1 -> gain_actBFV/1
  Sum/1 -> gain_actBFL/1
  Mux1/1 -> actBF/1
  Mux2/1 -> fbBF/1
  Demux1/3 -> Sum2/1
  Demux1/2 -> Sum1/1
  Demux1/1 -> Sum/1
  servoBFR/1 -> gainBFR/1
  servoBFP/1 -> gainBFP/1
  Sum6/1 -> Sum3/2, Mux2/4
  Sum7/1 -> Sum4/2, Mux2/5
  Demux/4 -> servoBFR/1
  Demux/5 -> servoBFP/1
  Demux1/4 -> Sum3/1
  Demux1/5 -> Sum4/1
  Sum3/1 -> gain_actBFR/1
  Sum4/1 -> gain_actBFP/1
  servoBFY/1 -> gainBFY/1
  Sum8/1 -> Sum5/2, Mux2/6
  Demux/6 -> servoBFY/1
  Sum5/1 -> gain_actBFY/1
  Demux1/6 -> Sum5/1
  gain_actBFV/1 -> Mux1/3
  gain_actBFY/1 -> Mux1/6
  gain_actBFR/1 -> Mux1/4
  gain_actBFT/1 -> Mux1/2
  gain_actBFL/1 -> Mux1/1
  gain_actBFP/1 -> Mux1/5
  servoHieBFR/1 -> gainHieBFR/1
  servoHieBFP/1 -> gainHieBFP/1
  servoHieBFY/1 -> gainHieBFY/1
  hieBF/1 -> Demux2/1
  gainBFR/1 -> Sum6/1
  gainBFP/1 -> Sum7/1
  gainBFY/1 -> Sum8/1
  gainHieBFR/1 -> Sum6/2
  gainHieBFP/1 -> Sum7/2
  gainHieBFY/1 -> Sum8/2
  Demux2/1 -> servoHieBFL/1
  Demux2/2 -> servoHieBFR/1
  Demux2/3 -> servoHieBFP/1
  Demux2/4 -> servoHieBFY/1
  servoHieBFL/1 -> gainHieBFL/1
  gainBFL/1 -> Sum9/1
  gainHieBFL/1 -> Sum9/2

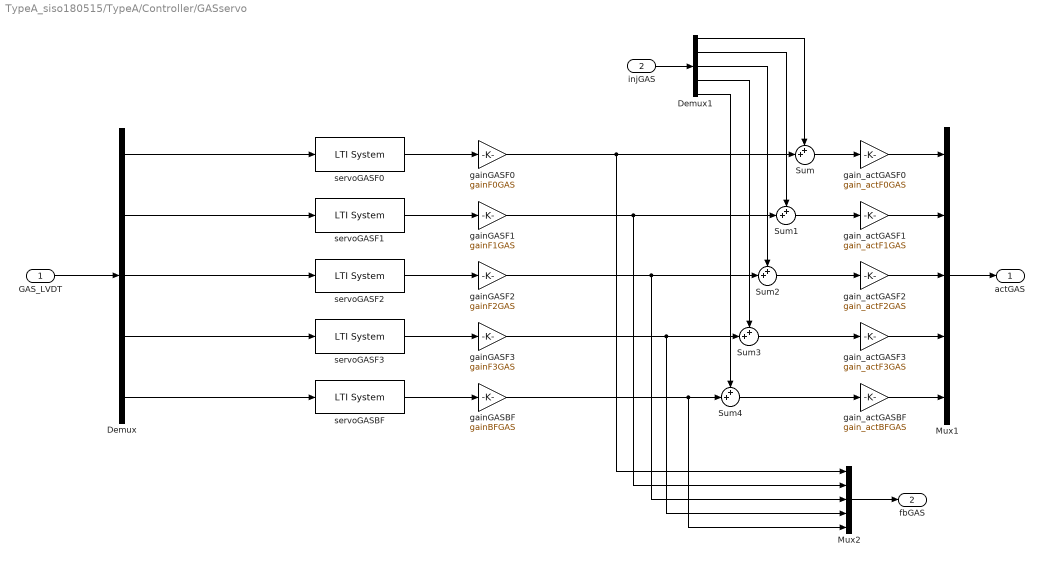
== system TypeA_siso180515/TypeA/Controller/GASservo ==
  GAS_LVDT : Inport
  injGAS : Inport  Port=2
  Demux : Demux  Outputs=5
  Demux1 : Demux  Outputs=5
  Mux1 : Mux  Inputs=5
  Mux2 : Mux  Inputs=5
  Sum{,1..4} (5 alike) : Sum  Inputs=++|
  gainGASBF : Gain  Gain=gainBFGAS
  gainGASF0 : Gain  Gain=gainF0GAS
  gainGASF1 : Gain  Gain=gainF1GAS
  gainGASF2 : Gain  Gain=gainF2GAS
  gainGASF3 : Gain  Gain=gainF3GAS
  gain_actGASBF : Gain  Gain=gain_actBFGAS
  gain_actGASF0 : Gain  Gain=gain_actF0GAS
  gain_actGASF1 : Gain  Gain=gain_actF1GAS
  gain_actGASF2 : Gain  Gain=gain_actF2GAS
  gain_actGASF3 : Gain  Gain=gain_actF3GAS
  servoGASBF : cstblocks/LTI System  sys=servoBFGAS  IC=[]
  servoGASF0 : cstblocks/LTI System  sys=servoF0GAS  IC=[]
  servoGASF1 : cstblocks/LTI System  sys=servoF1GAS  IC=[]
  servoGASF2 : cstblocks/LTI System  sys=servoF2GAS  IC=[]
  servoGASF3 : cstblocks/LTI System  sys=servoF3GAS  IC=[]
  actGAS : Outport
  fbGAS : Outport  Port=2
  wires:
  GAS_LVDT/1 -> Demux/1
  servoGASF0/1 -> gainGASF0/1
  servoGASF1/1 -> gainGASF1/1
  servoGASF2/1 -> gainGASF2/1
  Demux/1 -> servoGASF0/1
  Demux/2 -> servoGASF1/1
  Demux/3 -> servoGASF2/1
  gainGASF0/1 -> Sum/2, Mux2/1
  gainGASF1/1 -> Sum1/2, Mux2/2
  gainGASF2/1 -> Sum2/2, Mux2/3
  injGAS/1 -> Demux1/1
  Sum1/1 -> gain_actGASF1/1
  Sum2/1 -> gain_actGASF2/1
  Sum/1 -> gain_actGASF0/1
  Mux1/1 -> actGAS/1
  Mux2/1 -> fbGAS/1
  Demux1/3 -> Sum2/1
  Demux1/2 -> Sum1/1
  Demux1/1 -> Sum/1
  servoGASF3/1 -> gainGASF3/1
  servoGASBF/1 -> gainGASBF/1
  gainGASF3/1 -> Sum3/2, Mux2/4
  gainGASBF/1 -> Sum4/2, Mux2/5
  Demux/4 -> servoGASF3/1
  Demux/5 -> servoGASBF/1
  Demux1/4 -> Sum3/1
  Demux1/5 -> Sum4/1
  Sum3/1 -> gain_actGASF3/1
  Sum4/1 -> gain_actGASBF/1
  gain_actGASF0/1 -> Mux1/1
  gain_actGASF2/1 -> Mux1/3
  gain_actGASF1/1 -> Mux1/2
  gain_actGASF3/1 -> Mux1/4
  gain_actGASBF/1 -> Mux1/5

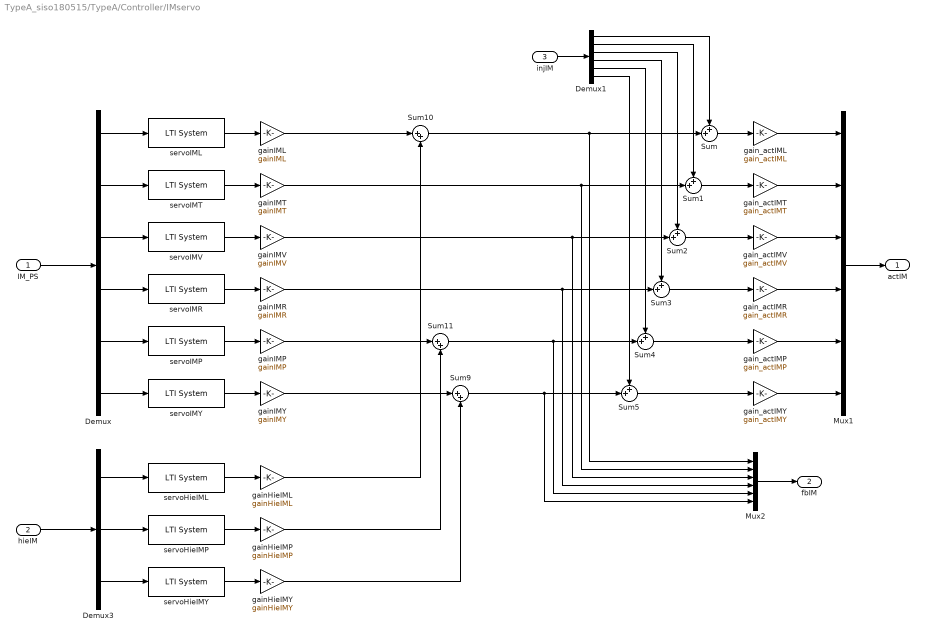
== system TypeA_siso180515/TypeA/Controller/IMservo ==
  IM_PS : Inport
  hieIM : Inport  Port=2
  injIM : Inport  Port=3
  Demux : Demux  Outputs=6
  Demux1 : Demux  Outputs=6
  Demux3 : Demux  Outputs=3
  Mux1 : Mux  Inputs=6
  Mux2 : Mux  Inputs=6
  Sum{,1..5} (6 alike) : Sum  Inputs=++|
  Sum10 : Sum  Inputs=|++
  Sum11 : Sum  Inputs=|++
  Sum9 : Sum  Inputs=|++
  gainHieIML : Gain  Gain=gainHieIML
  gainHieIMP : Gain  Gain=gainHieIMP
  gainHieIMY : Gain  Gain=gainHieIMY
  gainIML : Gain  Gain=gainIML
  gainIMP : Gain  Gain=gainIMP
  gainIMR : Gain  Gain=gainIMR
  gainIMT : Gain  Gain=gainIMT
  gainIMV : Gain  Gain=gainIMV
  gainIMY : Gain  Gain=gainIMY
  gain_actIML : Gain  Gain=gain_actIML
  gain_actIMP : Gain  Gain=gain_actIMP
  gain_actIMR : Gain  Gain=gain_actIMR
  gain_actIMT : Gain  Gain=gain_actIMT
  gain_actIMV : Gain  Gain=gain_actIMV
  gain_actIMY : Gain  Gain=gain_actIMY
  servoHieIML : cstblocks/LTI System  sys=servoHieIML  IC=[]
  servoHieIMP : cstblocks/LTI System  sys=servoHieIMP  IC=[]
  servoHieIMY : cstblocks/LTI System  sys=servoHieIMY  IC=[]
  servoIML : cstblocks/LTI System  sys=servoIML  IC=[]
  servoIMP : cstblocks/LTI System  sys=servoIMP  IC=[]
  servoIMR : cstblocks/LTI System  sys=servoIMR  IC=[]
  servoIMT : cstblocks/LTI System  sys=servoIMT  IC=[]
  servoIMV : cstblocks/LTI System  sys=servoIMV  IC=[]
  servoIMY : cstblocks/LTI System  sys=servoIMY  IC=[]
  actIM : Outport
  fbIM : Outport  Port=2
  wires:
  IM_PS/1 -> Demux/1
  servoIML/1 -> gainIML/1
  servoIMT/1 -> gainIMT/1
  servoIMV/1 -> gainIMV/1
  Demux/1 -> servoIML/1
  Demux/2 -> servoIMT/1
  Demux/3 -> servoIMV/1
  Sum10/1 -> Sum/2, Mux2/1
  gainIMT/1 -> Sum1/2, Mux2/2
  gainIMV/1 -> Sum2/2, Mux2/3
  injIM/1 -> Demux1/1
  Sum1/1 -> gain_actIMT/1
  Sum2/1 -> gain_actIMV/1
  Sum/1 -> gain_actIML/1
  Mux1/1 -> actIM/1
  Mux2/1 -> fbIM/1
  Demux1/3 -> Sum2/1
  Demux1/2 -> Sum1/1
  Demux1/1 -> Sum/1
  servoIMR/1 -> gainIMR/1
  servoIMP/1 -> gainIMP/1
  gainIMR/1 -> Sum3/2, Mux2/4
  Sum11/1 -> Sum4/2, Mux2/5
  Demux/4 -> servoIMR/1
  Demux/5 -> servoIMP/1
  Demux1/4 -> Sum3/1
  Demux1/5 -> Sum4/1
  Sum3/1 -> gain_actIMR/1
  Sum4/1 -> gain_actIMP/1
  servoIMY/1 -> gainIMY/1
  Sum9/1 -> Sum5/2, Mux2/6
  Demux/6 -> servoIMY/1
  Sum5/1 -> gain_actIMY/1
  Demux1/6 -> Sum5/1
  gain_actIMV/1 -> Mux1/3
  gain_actIMY/1 -> Mux1/6
  gain_actIMR/1 -> Mux1/4
  gain_actIMT/1 -> Mux1/2
  gain_actIML/1 -> Mux1/1
  gain_actIMP/1 -> Mux1/5
  servoHieIML/1 -> gainHieIML/1
  servoHieIMP/1 -> gainHieIMP/1
  servoHieIMY/1 -> gainHieIMY/1
  hieIM/1 -> Demux3/1
  Demux3/1 -> servoHieIML/1
  Demux3/2 -> servoHieIMP/1
  Demux3/3 -> servoHieIMY/1
  gainIML/1 -> Sum10/1
  gainIMP/1 -> Sum11/1
  gainHieIML/1 -> Sum10/2
  gainHieIMP/1 -> Sum11/2
  gainHieIMY/1 -> Sum9/2
  gainIMY/1 -> Sum9/1

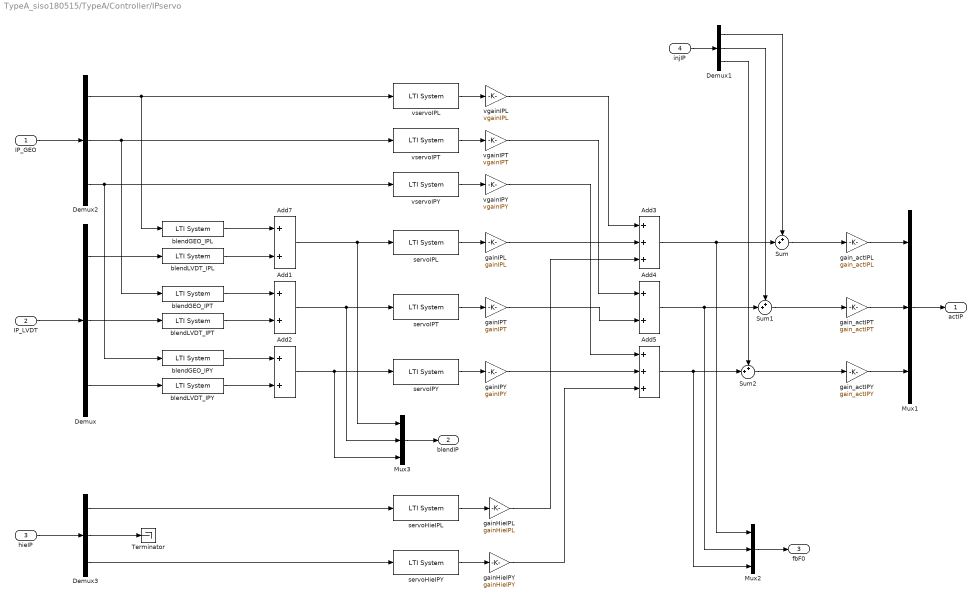
== system TypeA_siso180515/TypeA/Controller/IPservo ==
  IP_GEO : Inport
  IP_LVDT : Inport  Port=2
  hieIP : Inport  Port=3
  injIP : Inport  Port=4
  Add{1..2,4,7} (4 alike) : Sum
  Add3 : Sum  Inputs=+++
  Add5 : Sum  Inputs=+++
  Demux{,1..3} (4 alike) : Demux  Outputs=3
  Mux1 : Mux  Inputs=3
  Mux2 : Mux  Inputs=3
  Mux3 : Mux  Inputs=3
  Sum : Sum  Inputs=++|
  Sum1 : Sum  Inputs=++|
  Sum2 : Sum  Inputs=++|
  Terminator : Terminator
  blendGEO_IPL : cstblocks/LTI System  sys=blendGEO_IPL  IC=[]
  blendGEO_IPT : cstblocks/LTI System  sys=blendGEO_IPT  IC=[]
  blendGEO_IPY : cstblocks/LTI System  sys=blendGEO_IPY  IC=[]
  blendLVDT_IPL : cstblocks/LTI System  sys=blendLVDT_IPL  IC=[]
  blendLVDT_IPT : cstblocks/LTI System  sys=blendLVDT_IPT  IC=[]
  blendLVDT_IPY : cstblocks/LTI System  sys=blendLVDT_IPY  IC=[]
  gainHieIPL : Gain  Gain=gainHieIPL
  gainHieIPY : Gain  Gain=gainHieIPY
  gainIPL : Gain  Gain=gainIPL
  gainIPT : Gain  Gain=gainIPT
  gainIPY : Gain  Gain=gainIPY
  gain_actIPL : Gain  Gain=gain_actIPL
  gain_actIPT : Gain  Gain=gain_actIPT
  gain_actIPY : Gain  Gain=gain_actIPY
  servoHieIPL : cstblocks/LTI System  sys=servoHieIPL  IC=[]
  servoHieIPY : cstblocks/LTI System  sys=servoHieIPY  IC=[]
  servoIPL : cstblocks/LTI System  sys=servoIPL  IC=[]
  servoIPT : cstblocks/LTI System  sys=servoIPT  IC=[]
  servoIPY : cstblocks/LTI System  sys=servoIPY  IC=[]
  vgainIPL : Gain  Gain=vgainIPL
  vgainIPT : Gain  Gain=vgainIPT
  vgainIPY : Gain  Gain=vgainIPY
  vservoIPL : cstblocks/LTI System  sys=vservoIPL  IC=[]
  vservoIPT : cstblocks/LTI System  sys=vservoIPT  IC=[]
  vservoIPY : cstblocks/LTI System  sys=vservoIPY  IC=[]
  actIP : Outport
  blendIP : Outport  Port=2
  fbF0 : Outport  Port=3
  wires:
  IP_LVDT/1 -> Demux/1
  servoIPL/1 -> gainIPL/1
  servoIPT/1 -> gainIPT/1
  servoIPY/1 -> gainIPY/1
  Add3/1 -> Sum/2, Mux2/1
  Add4/1 -> Sum1/2, Mux2/2
  Add5/1 -> Sum2/2, Mux2/3
  injIP/1 -> Demux1/1
  Sum1/1 -> gain_actIPT/1
  Sum2/1 -> gain_actIPY/1
  Sum/1 -> gain_actIPL/1
  Mux1/1 -> actIP/1
  Mux2/1 -> fbF0/1
  Demux1/3 -> Sum2/1
  Demux1/2 -> Sum1/1
  Demux1/1 -> Sum/1
  gain_actIPT/1 -> Mux1/2
  gain_actIPL/1 -> Mux1/1
  gain_actIPY/1 -> Mux1/3
  Demux/2 -> blendLVDT_IPT/1
  Demux/3 -> blendLVDT_IPY/1
  Demux/1 -> blendLVDT_IPL/1
  IP_GEO/1 -> Demux2/1
  Demux2/2 -> vservoIPT/1, blendGEO_IPT/1
  Demux2/3 -> vservoIPY/1, blendGEO_IPY/1
  Demux2/1 -> vservoIPL/1, blendGEO_IPL/1
  Add7/1 -> Mux3/1, servoIPL/1
  Add1/1 -> Mux3/2, servoIPT/1
  Add2/1 -> Mux3/3, servoIPY/1
  blendGEO_IPL/1 -> Add7/1
  blendGEO_IPT/1 -> Add1/1
  blendGEO_IPY/1 -> Add2/1
  blendLVDT_IPL/1 -> Add7/2
  blendLVDT_IPT/1 -> Add1/2
  blendLVDT_IPY/1 -> Add2/2
  Mux3/1 -> blendIP/1
  vservoIPL/1 -> vgainIPL/1
  vservoIPT/1 -> vgainIPT/1
  vservoIPY/1 -> vgainIPY/1
  gainIPY/1 -> Add5/2
  gainIPT/1 -> Add4/2
  gainIPL/1 -> Add3/2
  vgainIPL/1 -> Add3/1
  vgainIPT/1 -> Add4/1
  vgainIPY/1 -> Add5/1
  servoHieIPL/1 -> gainHieIPL/1
  servoHieIPY/1 -> gainHieIPY/1
  hieIP/1 -> Demux3/1
  Demux3/1 -> servoHieIPL/1
  Demux3/3 -> servoHieIPY/1
  gainHieIPL/1 -> Add3/3
  gainHieIPY/1 -> Add5/3
  Demux3/2 -> Terminator/1

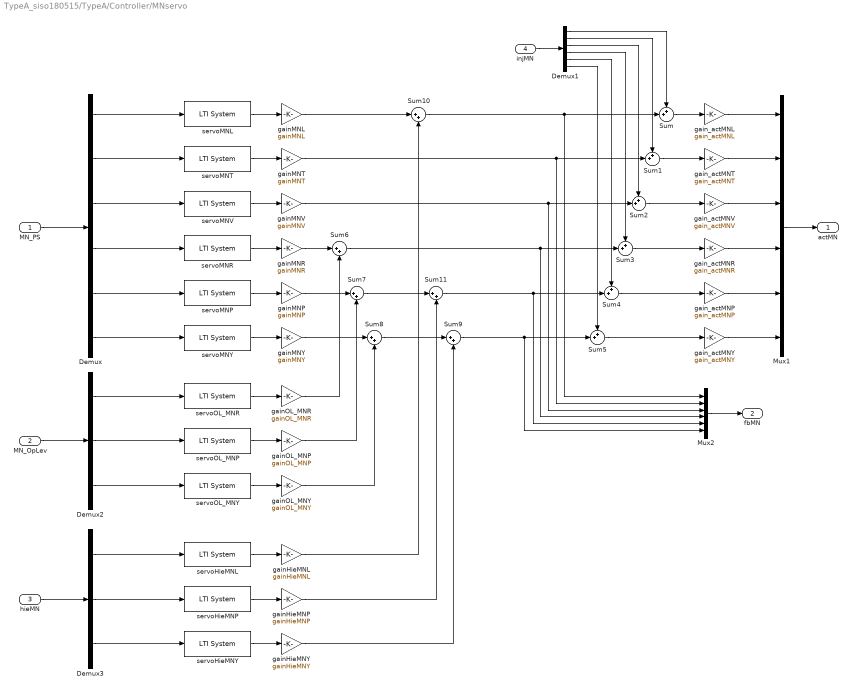
== system TypeA_siso180515/TypeA/Controller/MNservo ==
  MN_PS : Inport
  MN_OpLev : Inport  Port=2
  hieMN : Inport  Port=3
  injMN : Inport  Port=4
  Demux : Demux  Outputs=6
  Demux1 : Demux  Outputs=6
  Demux2 : Demux  Outputs=3
  Demux3 : Demux  Outputs=3
  Mux1 : Mux  Inputs=6
  Mux2 : Mux  Inputs=6
  Sum{,1..5} (6 alike) : Sum  Inputs=++|
  Sum{6..11} (6 alike) : Sum  Inputs=|++
  gainHieMNL : Gain  Gain=gainHieMNL
  gainHieMNP : Gain  Gain=gainHieMNP
  gainHieMNY : Gain  Gain=gainHieMNY
  gainMNL : Gain  Gain=gainMNL
  gainMNP : Gain  Gain=gainMNP
  gainMNR : Gain  Gain=gainMNR
  gainMNT : Gain  Gain=gainMNT
  gainMNV : Gain  Gain=gainMNV
  gainMNY : Gain  Gain=gainMNY
  gainOL_MNP : Gain  Gain=gainOL_MNP
  gainOL_MNR : Gain  Gain=gainOL_MNR
  gainOL_MNY : Gain  Gain=gainOL_MNY
  gain_actMNL : Gain  Gain=gain_actMNL
  gain_actMNP : Gain  Gain=gain_actMNP
  gain_actMNR : Gain  Gain=gain_actMNR
  gain_actMNT : Gain  Gain=gain_actMNT
  gain_actMNV : Gain  Gain=gain_actMNV
  gain_actMNY : Gain  Gain=gain_actMNY
  servoHieMNL : cstblocks/LTI System  sys=servoHieMNL  IC=[]
  servoHieMNP : cstblocks/LTI System  sys=servoHieMNP  IC=[]
  servoHieMNY : cstblocks/LTI System  sys=servoHieMNY  IC=[]
  servoMNL : cstblocks/LTI System  sys=servoMNL  IC=[]
  servoMNP : cstblocks/LTI System  sys=servoMNP  IC=[]
  servoMNR : cstblocks/LTI System  sys=servoMNR  IC=[]
  servoMNT : cstblocks/LTI System  sys=servoMNT  IC=[]
  servoMNV : cstblocks/LTI System  sys=servoMNV  IC=[]
  servoMNY : cstblocks/LTI System  sys=servoMNY  IC=[]
  servoOL_MNP : cstblocks/LTI System  sys=servoOL_MNP  IC=[]
  servoOL_MNR : cstblocks/LTI System  sys=servoOL_MNR  IC=[]
  servoOL_MNY : cstblocks/LTI System  sys=servoOL_MNY  IC=[]
  actMN : Outport
  fbMN : Outport  Port=2
  wires:
  MN_PS/1 -> Demux/1
  servoMNL/1 -> gainMNL/1
  servoMNT/1 -> gainMNT/1
  servoMNV/1 -> gainMNV/1
  Demux/1 -> servoMNL/1
  Demux/2 -> servoMNT/1
  Demux/3 -> servoMNV/1
  Sum10/1 -> Sum/2, Mux2/1
  gainMNT/1 -> Sum1/2, Mux2/2
  gainMNV/1 -> Sum2/2, Mux2/3
  injMN/1 -> Demux1/1
  Sum1/1 -> gain_actMNT/1
  Sum2/1 -> gain_actMNV/1
  Sum/1 -> gain_actMNL/1
  Mux1/1 -> actMN/1
  Mux2/1 -> fbMN/1
  Demux1/3 -> Sum2/1
  Demux1/2 -> Sum1/1
  Demux1/1 -> Sum/1
  servoMNR/1 -> gainMNR/1
  servoMNP/1 -> gainMNP/1
  Sum6/1 -> Sum3/2, Mux2/4
  Sum11/1 -> Sum4/2, Mux2/5
  Demux/4 -> servoMNR/1
  Demux/5 -> servoMNP/1
  Demux1/4 -> Sum3/1
  Demux1/5 -> Sum4/1
  Sum3/1 -> gain_actMNR/1
  Sum4/1 -> gain_actMNP/1
  servoMNY/1 -> gainMNY/1
  Sum9/1 -> Sum5/2, Mux2/6
  Demux/6 -> servoMNY/1
  Sum5/1 -> gain_actMNY/1
  Demux1/6 -> Sum5/1
  gain_actMNV/1 -> Mux1/3
  gain_actMNY/1 -> Mux1/6
  gain_actMNR/1 -> Mux1/4
  gain_actMNT/1 -> Mux1/2
  gain_actMNL/1 -> Mux1/1
  gain_actMNP/1 -> Mux1/5
  servoHieMNL/1 -> gainHieMNL/1
  servoHieMNP/1 -> gainHieMNP/1
  servoHieMNY/1 -> gainHieMNY/1
  servoOL_MNR/1 -> gainOL_MNR/1
  servoOL_MNP/1 -> gainOL_MNP/1
  servoOL_MNY/1 -> gainOL_MNY/1
  MN_OpLev/1 -> Demux2/1
  hieMN/1 -> Demux3/1
  Demux2/1 -> servoOL_MNR/1
  Demux2/2 -> servoOL_MNP/1
  Demux2/3 -> servoOL_MNY/1
  Demux3/1 -> servoHieMNL/1
  gainMNR/1 -> Sum6/1
  gainMNP/1 -> Sum7/1
  gainMNY/1 -> Sum8/1
  gainOL_MNR/1 -> Sum6/2
  gainOL_MNP/1 -> Sum7/2
  gainOL_MNY/1 -> Sum8/2
  gainMNL/1 -> Sum10/1
  Sum7/1 -> Sum11/1
  gainHieMNL/1 -> Sum10/2
  gainHieMNP/1 -> Sum11/2
  gainHieMNY/1 -> Sum9/2
  Sum8/1 -> Sum9/1
  Demux3/2 -> servoHieMNP/1
  Demux3/3 -> servoHieMNY/1

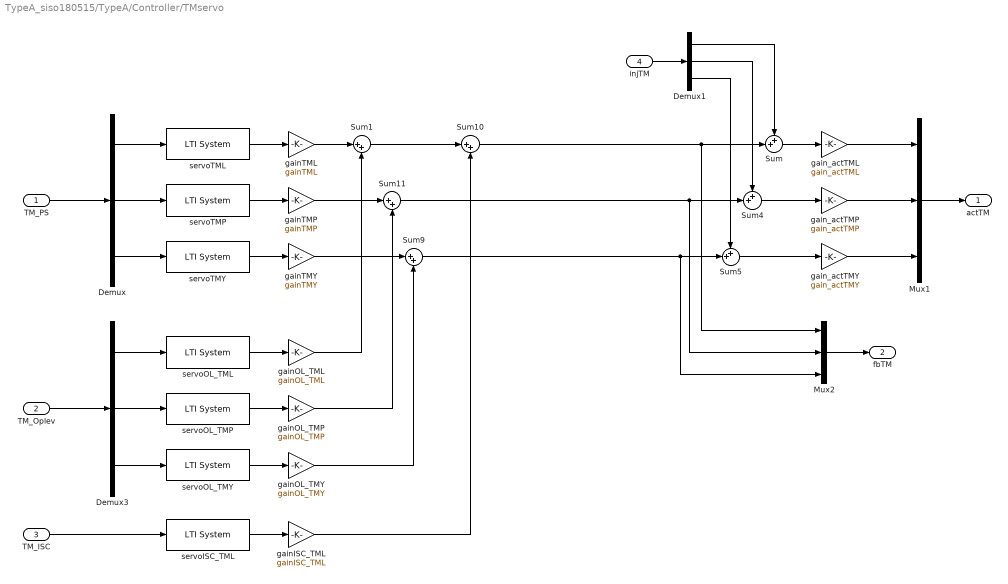
== system TypeA_siso180515/TypeA/Controller/TMservo ==
  TM_PS : Inport
  TM_Oplev : Inport  Port=2
  TM_ISC : Inport  Port=3
  injTM : Inport  Port=4
  Demux : Demux  Outputs=3
  Demux1 : Demux  Outputs=3
  Demux3 : Demux  Outputs=3
  Mux1 : Mux  Inputs=3
  Mux2 : Mux  Inputs=3
  Sum : Sum  Inputs=++|
  Sum{1,9..11} (4 alike) : Sum  Inputs=|++
  Sum4 : Sum  Inputs=++|
  Sum5 : Sum  Inputs=++|
  gainISC_TML : Gain  Gain=gainISC_TML
  gainOL_TML : Gain  Gain=gainOL_TML
  gainOL_TMP : Gain  Gain=gainOL_TMP
  gainOL_TMY : Gain  Gain=gainOL_TMY
  gainTML : Gain  Gain=gainTML
  gainTMP : Gain  Gain=gainTMP
  gainTMY : Gain  Gain=gainTMY
  gain_actTML : Gain  Gain=gain_actTML
  gain_actTMP : Gain  Gain=gain_actTMP
  gain_actTMY : Gain  Gain=gain_actTMY
  servoISC_TML : cstblocks/LTI System  sys=servoISC_TML  IC=[]
  servoOL_TML : cstblocks/LTI System  sys=servoOL_TML  IC=[]
  servoOL_TMP : cstblocks/LTI System  sys=servoOL_TMP  IC=[]
  servoOL_TMY : cstblocks/LTI System  sys=servoOL_TMY  IC=[]
  servoTML : cstblocks/LTI System  sys=servoTML  IC=[]
  servoTMP : cstblocks/LTI System  sys=servoTMP  IC=[]
  servoTMY : cstblocks/LTI System  sys=servoTMY  IC=[]
  actTM : Outport
  fbTM : Outport  Port=2
  wires:
  TM_PS/1 -> Demux/1
  servoTML/1 -> gainTML/1
  Demux/1 -> servoTML/1
  Sum10/1 -> Sum/2, Mux2/1
  injTM/1 -> Demux1/1
  Sum/1 -> gain_actTML/1
  Mux1/1 -> actTM/1
  Mux2/1 -> fbTM/1
  Demux1/1 -> Sum/1
  servoTMP/1 -> gainTMP/1
  Sum11/1 -> Mux2/2, Sum4/2
  Sum4/1 -> gain_actTMP/1
  servoTMY/1 -> gainTMY/1
  Sum9/1 -> Mux2/3, Sum5/2
  Sum5/1 -> gain_actTMY/1
  gain_actTML/1 -> Mux1/1
  servoOL_TMP/1 -> gainOL_TMP/1
  servoOL_TMY/1 -> gainOL_TMY/1
  TM_Oplev/1 -> Demux3/1
  Demux3/2 -> servoOL_TMP/1
  Demux3/3 -> servoOL_TMY/1
  gainTML/1 -> Sum1/1
  gainTMP/1 -> Sum11/1
  gainOL_TMP/1 -> Sum11/2
  gainOL_TMY/1 -> Sum9/2
  gainTMY/1 -> Sum9/1
  Demux/2 -> servoTMP/1
  Demux/3 -> servoTMY/1
  Demux1/2 -> Sum4/1
  Demux1/3 -> Sum5/1
  gain_actTMP/1 -> Mux1/2
  gain_actTMY/1 -> Mux1/3
  servoISC_TML/1 -> gainISC_TML/1
  TM_ISC/1 -> servoISC_TML/1
  gainISC_TML/1 -> Sum10/2
  Demux3/1 -> servoOL_TML/1
  Sum1/1 -> Sum10/1
  gainOL_TML/1 -> Sum1/2
  servoOL_TML/1 -> gainOL_TML/1

== system TypeA_siso180515/TypeA/Controller/sum ==
  localTM : Inport
  globalISC : Inport  Port=2
  Demux4 : Demux  Outputs=3
  Mux3 : Mux  Inputs=3
  Sum : Sum  Inputs=++|
  toUpperStage : Outport
  wires:
  localTM/1 -> Demux4/1
  Mux3/1 -> toUpperStage/1
  Demux4/1 -> Sum/2  "L"
  Demux4/2 -> Mux3/2  "P"
  Demux4/3 -> Mux3/3  "Y"
  globalISC/1 -> Sum/1
  Sum/1 -> Mux3/1

== system TypeA_siso180515/TypeA/Controller/sum1 ==
  fromPF : Inport
  fromTM : Inport  Port=2
  Demux1 : Demux  Outputs=3
  Demux4 : Demux  Outputs=3
  Mux3 : Mux
  Sum : Sum  Inputs=++|
  Sum1 : Sum  Inputs=++|
  toBF : Outport
  wires:
  fromTM/1 -> Demux4/1
  Mux3/1 -> toBF/1
  Demux4/2 -> Sum/2  "P"
  Demux4/3 -> Sum1/2  "Y"
  fromPF/1 -> Demux1/1
  Sum1/1 -> Mux3/4
  Demux4/1 -> Mux3/1  "L"
  Demux1/2 -> Sum/1  "P"
  Demux1/3 -> Sum1/1  "Y"
  Sum/1 -> Mux3/3
  Demux1/1 -> Mux3/2  "R"
